simulink model "NyModel"  (R2020b)
settings: Solver=VariableStepAuto  StartTime=0.0  StopTime=10  RelTol=1e-3
settings Model: Creator=jonas  LastModifiedBy=jonas
settings SolverCC: ZeroCrossAlgorithm=Adaptive
settings DebuggingCC: IgnoredZcDiagnostic=none

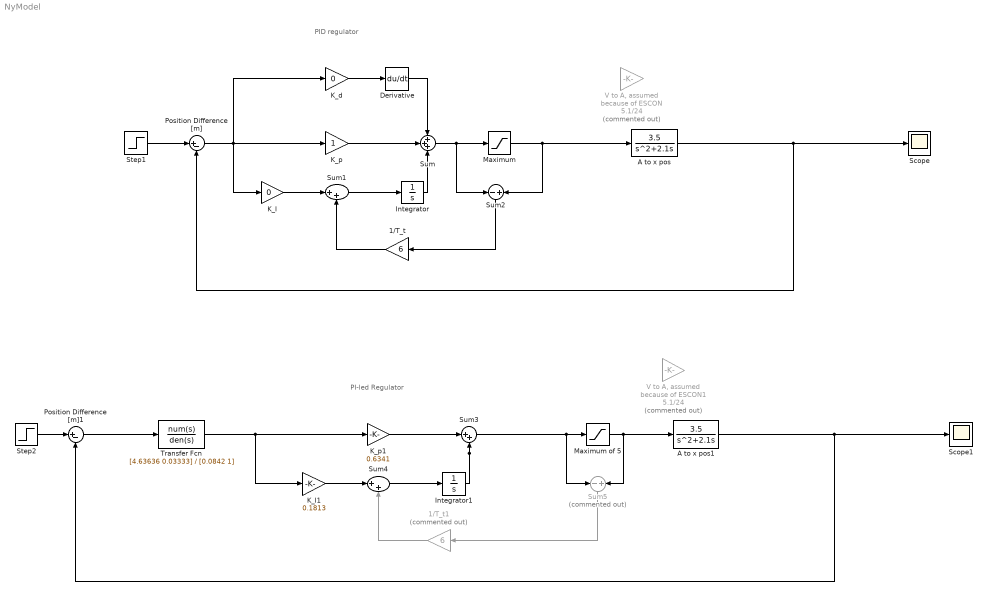
== system NyModel ==
  note: PI-led Regulator
  note: PID regulator
  1/T_t : Gain  Gain=6
  1/T_t1 : Gain  Commented=on  Gain=6
  A to x pos : TransferFcn  Numerator=[3.5]  Denominator=[1 2.1 0]
  A to x pos1 : TransferFcn  Numerator=[3.5]  Denominator=[1 2.1 0]
  Derivative : Derivative
  Integrator : Integrator
  Integrator1 : Integrator
  K_I : Gain  Gain=0
  K_I1 : Gain  Gain=0.1813
  K_d : Gain  Gain=0
  K_p : Gain
  K_p1 : Gain  Gain=0.6341
  Maximum : Saturate  UpperLimit=5  LowerLimit=-5
  Maximum of 5 : Saturate  UpperLimit=5  LowerLimit=-5
  Position Difference [m] : Sum  Inputs=|+-
  Position Difference [m]1 : Sum  Inputs=|+-
  Scope : Scope
  Scope1 : Scope
  Step1 : Step  Time=0  SampleTime=0
  Step2 : Step  Time=0  SampleTime=0
  Sum : Sum  Inputs=+++
  Sum1 : Sum  Inputs=|++
  Sum2 : Sum  Inputs=-+
  Sum3 : Sum  Inputs=|++
  Sum4 : Sum  Inputs=|++
  Sum5 : Sum  Commented=on  Inputs=-+
  Transfer Fcn : TransferFcn  Numerator=[4.63636 0.03333]  Denominator=[0.0842 1]
  "V to A, assumed because of ESCON" : Gain  Commented=on  Gain=5.1/24
  "V to A, assumed because of ESCON1" : Gain  Commented=on  Gain=5.1/24
  wires:
  Step1/1 -> Position Difference [m]/1
  A to x pos/1 -> Scope/1, Position Difference [m]/2
  K_d/1 -> Derivative/1
  Derivative/1 -> Sum/1
  K_p/1 -> Sum/2
  K_I/1 -> Sum1/1
  Sum1/1 -> Integrator/1
  Integrator/1 -> Sum/3
  Sum/1 -> Sum2/1, Maximum/1
  Sum2/1 -> 1/T_t/1
  1/T_t/1 -> Sum1/2
  Position Difference [m]/1 -> K_I/1, K_d/1, K_p/1
  Maximum/1 -> A to x pos/1, Sum2/2
  Step2/1 -> Position Difference [m]1/1
  Maximum of 5/1 -> A to x pos1/1, Sum5/2
  1/T_t1/1 -> Sum4/2
  Integrator1/1 -> Sum3/2
  Sum4/1 -> Integrator1/1
  Sum5/1 -> 1/T_t1/1
  K_I1/1 -> Sum4/1
  A to x pos1/1 -> Scope1/1, Position Difference [m]1/2
  Sum3/1 -> Sum5/1, Maximum of 5/1
  K_p1/1 -> Sum3/1
  Position Difference [m]1/1 -> Transfer Fcn/1
  Transfer Fcn/1 -> K_I1/1, K_p1/1
